simulink subsystem "Servo_Block"  (R2022b)
settings: Solver=VariableStepAuto  StartTime=0.0  StopTime=10.0  RelTol=1e-3
values from neighbouring files (symbols this model uses):
  alpha0 = ones(1,6) * servoCalc(P_default(:,1),b(:,1),sqrt(l0_squared),s,a,beta(1))    [StewartPlatformEqs.m]    (also in StewartPlatformEqs_JointAngles.m; StewartPlatformEqs_alpha.m; runSimulation.m = alpha0')
  DEN = [servoTimeConstant 1]    [runSimulation.m]
libraries: simulink_extras x6
settings Model: Creator=wiche  LastModifiedBy=peter
settings OptimizationCC: ReuseModelBlockBuffer=on

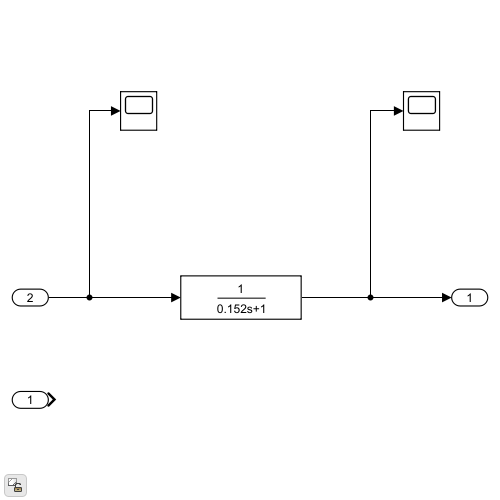
[thumbnail: Simulink's stored preview of the top-level diagram]
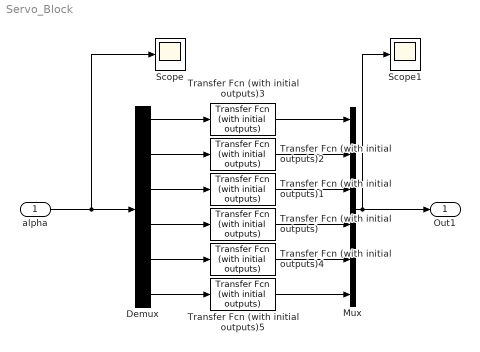
== system Servo_Block ==
  alpha : Inport
  Demux : Demux  Outputs=6
  Mux : Mux  Inputs=6
  Scope : Scope
  Scope1 : Scope
  Transfer Fcn (with initial outputs) : simulink_extras/Additional Linear/Transfer Fcn (with initial outputs)  N=[1]  D=DEN  Y0=alpha0(4)  U0=0
  Transfer Fcn (with initial outputs)1 : simulink_extras/Additional Linear/Transfer Fcn (with initial outputs)  N=[1]  D=DEN  Y0=alpha0(3)  U0=0
  Transfer Fcn (with initial outputs)2 : simulink_extras/Additional Linear/Transfer Fcn (with initial outputs)  N=[1]  D=DEN  Y0=alpha0(2)  U0=0
  Transfer Fcn (with initial outputs)3 : simulink_extras/Additional Linear/Transfer Fcn (with initial outputs)  N=[1]  D=DEN  Y0=alpha0(1)  U0=0
  Transfer Fcn (with initial outputs)4 : simulink_extras/Additional Linear/Transfer Fcn (with initial outputs)  N=[1]  D=DEN  Y0=alpha0(5)  U0=0
  Transfer Fcn (with initial outputs)5 : simulink_extras/Additional Linear/Transfer Fcn (with initial outputs)  N=[1]  D=DEN  Y0=alpha0(6)  U0=0
  Out1 : Outport
  wires:
  alpha/1 -> Demux/1, Scope/1
  Mux/1 -> Scope1/1, Out1/1
  Demux/4 -> Transfer Fcn (with initial outputs)/1
  Transfer Fcn (with initial outputs)/1 -> Mux/4
  Transfer Fcn (with initial outputs)1/1 -> Mux/3
  Demux/3 -> Transfer Fcn (with initial outputs)1/1
  Transfer Fcn (with initial outputs)2/1 -> Mux/2
  Demux/2 -> Transfer Fcn (with initial outputs)2/1
  Transfer Fcn (with initial outputs)3/1 -> Mux/1
  Demux/1 -> Transfer Fcn (with initial outputs)3/1
  Transfer Fcn (with initial outputs)4/1 -> Mux/5
  Demux/5 -> Transfer Fcn (with initial outputs)4/1
  Transfer Fcn (with initial outputs)5/1 -> Mux/6
  Demux/6 -> Transfer Fcn (with initial outputs)5/1
